simulink model "sm"  (R2017b)
settings: Solver=VariableStepAuto  StartTime=0.0  StopTime=10.0  RelTol=1e-3
undefined symbols (not defined in the file or in its folder): A, Ak, B, Bk, C, Ck, D, Dk, DT, init_sm, initk, ThetaCo_init, ThetaCo_step, ZCo_init, ZCo_step
settings Model: Creator=lefort@sirehna.com  LastModifiedBy=lefort
settings OptimizationCC: LifeSpan=inf
settings DebuggingCC: SFExecutionAtInitializationDiag=none
settings CodeAppCC: StateflowObjectComments=on

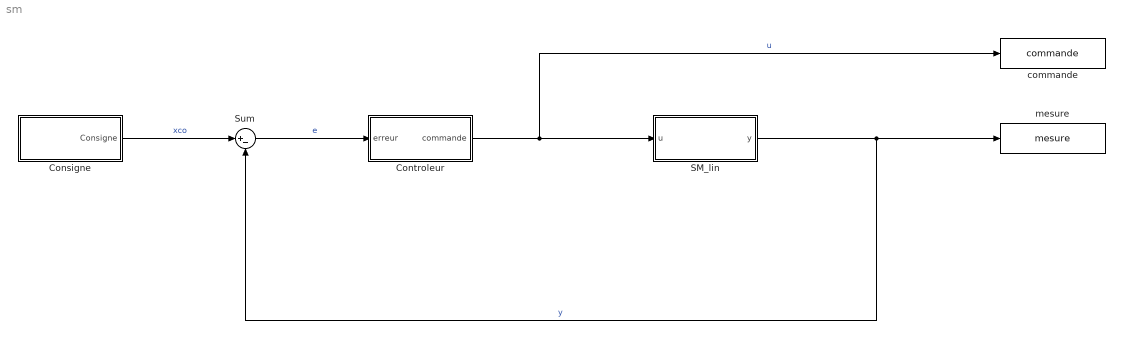
== system sm ==
  Consigne : Subsystem
  Controleur : Subsystem
  SM_lin : Subsystem
  Sum : Sum  Inputs=|+-
  commande : ToWorkspace  VariableName=commande  SaveFormat=Timeseries  SampleTime=-1
  mesure : ToWorkspace  VariableName=mesure  SaveFormat=Timeseries  SampleTime=-1
  wires:
  SM_lin/1(y) -> Sum/2, mesure/1  "y"
  Consigne/1(Consigne) -> Sum/1  "xco"
  Sum/1 -> Controleur/1(erreur)  "e"
  Controleur/1(commande) -> commande/1, SM_lin/1(u)  "u"

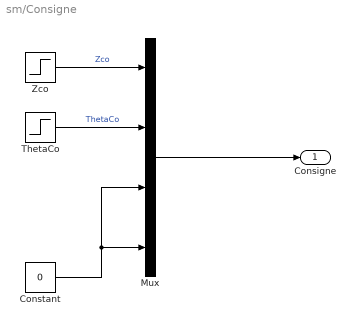
== system sm/Consigne ==
  Constant : Constant  Value=0
  Mux : Mux
  ThetaCo : Step  Time=DT  Before=ThetaCo_init  After=ThetaCo_step  SampleTime=DT
  Zco : Step  Time=DT  Before=ZCo_init  After=ZCo_step  SampleTime=DT
  Consigne : Outport
  wires:
  Mux/1 -> Consigne/1
  Constant/1 -> Mux/4, Mux/3
  Zco/1 -> Mux/1  "Zco"
  ThetaCo/1 -> Mux/2  "ThetaCo"

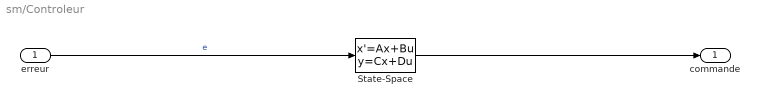
== system sm/Controleur ==
  erreur : Inport
  State-Space : StateSpace  A=Ak  B=Bk  C=Ck  D=Dk  InitialCondition=initk
  commande : Outport
  wires:
  erreur/1 -> State-Space/1  "e"
  State-Space/1 -> commande/1

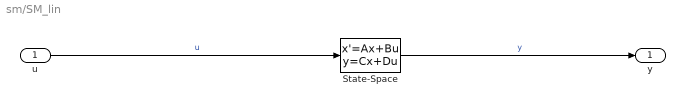
== system sm/SM_lin ==
  u : Inport
  State-Space : StateSpace  A=A  B=B  C=C  D=D  InitialCondition=init_sm
  y : Outport
  wires:
  State-Space/1 -> y/1  "y"
  u/1 -> State-Space/1  "u"
